simulink model "DateTimeAssemble_test"  (R2013a)
settings: Solver=ode3  StartTime=0.0  StopTime=200  FixedStep=0.001  RelTol=1e-3
libraries: simulink_extras x2, PTC_MBDS_LIB x1
settings Model: Creator=kyle.willis  LastModifiedBy=kyle.willis
settings OptimizationCC: InlineParams=on

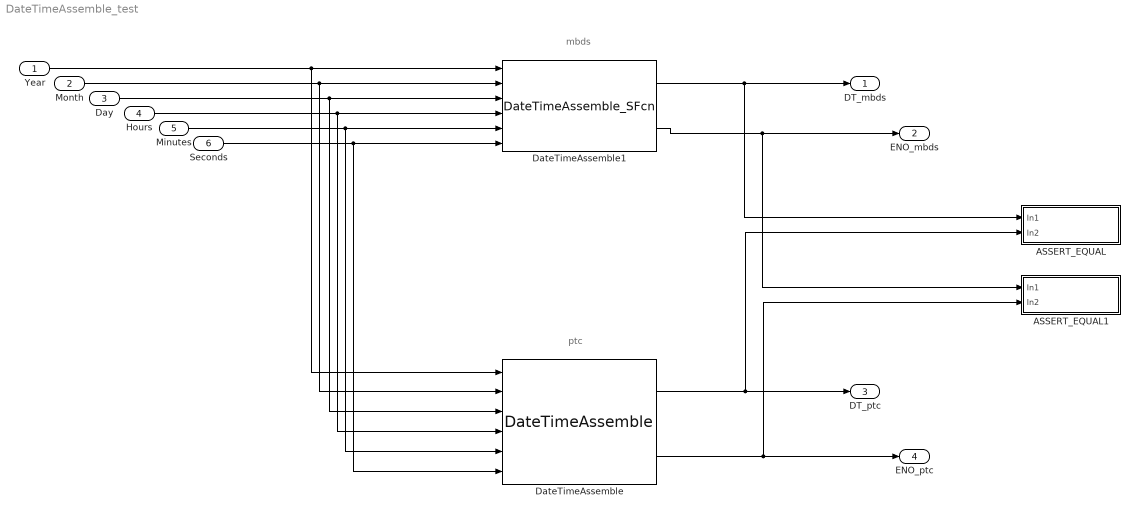
== system DateTimeAssemble_test ==
  note: ptc
  note: mbds
  Year : Inport
  Month : Inport  Port=2
  Day : Inport  Port=3
  Hours : Inport  Port=4
  Minutes : Inport  Port=5
  Seconds : Inport  Port=6
  ASSERT_EQUAL : Subsystem
  ASSERT_EQUAL1 : Subsystem
  DateTimeAssemble : PTC_MBDS_LIB/MBDS Standard Library/Extended Operations/Date & Time Operations/Date & Time Conversions/DateTimeAssemble  ENO_Enabled=on  PTC_MBDS_BlockVersion=5.40  PTC_BlockType=PTC_MBDS_DateTimeAssemble
  DateTimeAssemble1 : S-Function  InitFcn=|  FunctionName=DateTimeAssemble_SFcn  Parameters=boolean(ENO_Enabled)  EnableBusSupport=off  mask(DateTimeAssemble){MBDS_LibraryBlock=on, ENO_Enabled=on, MBDS_BlockVersion=05.41}
      | if(exist('MBDS_BlockCallback', 'file'))
      |    MBDS_BlockCallback('Update', gcb);  
      | end
      mask prompts: MBDS_LibraryBlock "MBDS Library Block"; ENO_Enabled "Show ENO port"; MBDS_BlockVersion "Block version:"
      mask help: Assembles a date_time signal from individual date and time components. The input values are restricted to their ranges (refer to the block help). If an input is out of range the ENO output is set to false.
      mask init:
      | MBDS_BlockCallback('Copy', gcb);     
      | maskdisplay = 'disp(sprintf(''Date Time\nAssemble''))';
      | maskdisplay = [maskdisplay 10 'port_label(''input'', 1, ''Year'')' 10];
      | maskdisplay = [maskdisplay 'port_label(''input'', 2, ''Month'')' 10];
      | maskdisplay = [maskdisplay 'port_label(''input'', 3, ''Day'')' 10];
      | maskdisplay = [maskdisplay 'port_label(''input'', 4, ''Hours'')' 10];
      | maskdisplay = [maskdisplay 'port_label(''input'', 5, ''Minutes'')' 10];
      | maskdisplay = [maskdisplay 'port_label(''input'', 6, ''Seconds'')' 10];
      | maskdisplay = [maskdisplay 'port_label(''output'', 1, ''DT'')' 10];
      | if(ENO_Enabled)
      |     maskdisplay = [maskdisplay 'port_label(''output'', 2, ''ENO'')' 10];
      | end
      | set_param(gcbh, 'maskdisplay', maskdisplay)
      mask Help: eval(['open([workdir(''RT_Dir:''),''\Host\Library\Blockset\Help\'',get_param(gcb,''MaskType''),''.html''])']);
      mask Display:
      | disp(sprintf('Date Time\nAssemble'))
      | port_label('input', 1, 'Year')
      | port_label('input', 2, 'Month')
      | port_label('input', 3, 'Day')
      | port_label('input', 4, 'Hours')
      | port_label('input', 5, 'Minutes')
      | port_label('input', 6, 'Seconds')
      | port_label('output', 1, 'DT')
      | port_label('output', 2, 'ENO')
  DT_mbds : Outport
  ENO_mbds : Outport  Port=2
  DT_ptc : Outport  Port=3
  ENO_ptc : Outport  Port=4
  wires:
  DateTimeAssemble/1 -> ASSERT_EQUAL/2(In2), DT_ptc/1
  DateTimeAssemble/2 -> ASSERT_EQUAL1/2(In2), ENO_ptc/1
  DateTimeAssemble1/1 -> ASSERT_EQUAL/1(In1), DT_mbds/1
  DateTimeAssemble1/2 -> ASSERT_EQUAL1/1(In1), ENO_mbds/1
  Year/1 -> DateTimeAssemble/1, DateTimeAssemble1/1
  Month/1 -> DateTimeAssemble1/2, DateTimeAssemble/2
  Day/1 -> DateTimeAssemble1/3, DateTimeAssemble/3
  Hours/1 -> DateTimeAssemble1/4, DateTimeAssemble/4
  Minutes/1 -> DateTimeAssemble1/5, DateTimeAssemble/5
  Seconds/1 -> DateTimeAssemble1/6, DateTimeAssemble/6

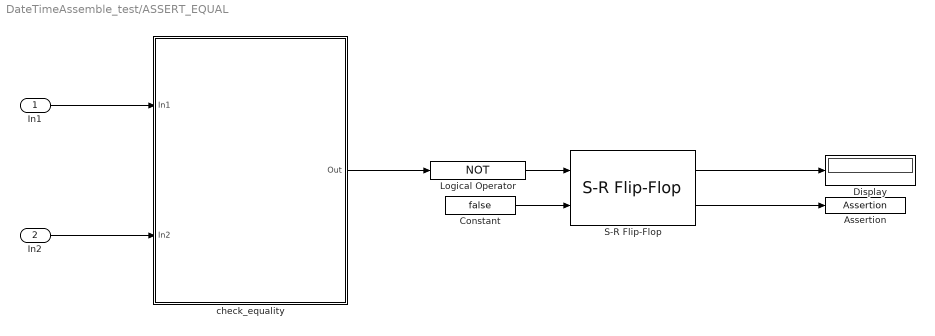
== system DateTimeAssemble_test/ASSERT_EQUAL ==
  In1 : Inport
  In2 : Inport  Port=2
  Assertion : Assertion
  Constant : Constant  Value=false
  Display : Display
  Logical Operator : Logic  Operator=NOT  AllPortsSameDT=off  OutDataTypeStr=boolean
  S-R Flip-Flop : simulink_extras/Flip Flops/S-R Flip-Flop  initial_condition=0
  check_equality : MATLAB Function  TreatAsAtomicUnit=on
  wires:
  S-R Flip-Flop/1 -> Display/1
  check_equality/1(Out) -> Logical Operator/1
  Constant/1 -> S-R Flip-Flop/2
  S-R Flip-Flop/2 -> Assertion/1
  In2/1 -> check_equality/2(In2)
  In1/1 -> check_equality/1(In1)
  Logical Operator/1 -> S-R Flip-Flop/1

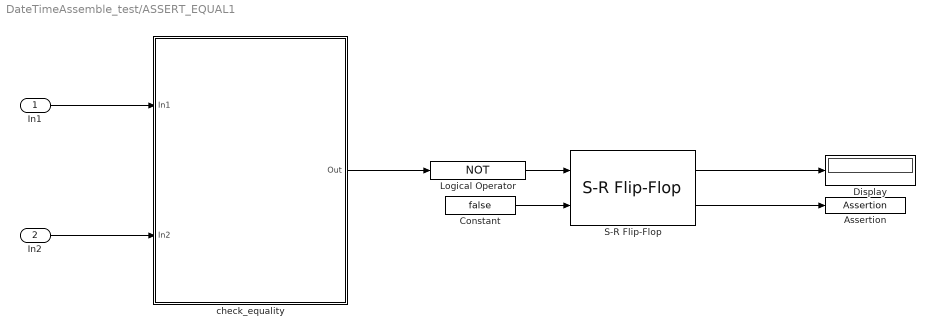
== system DateTimeAssemble_test/ASSERT_EQUAL1 ==
  In1 : Inport
  In2 : Inport  Port=2
  Assertion : Assertion
  Constant : Constant  Value=false
  Display : Display
  Logical Operator : Logic  Operator=NOT  AllPortsSameDT=off  OutDataTypeStr=boolean
  S-R Flip-Flop : simulink_extras/Flip Flops/S-R Flip-Flop  initial_condition=0
  check_equality : MATLAB Function  TreatAsAtomicUnit=on
  wires:
  Logical Operator/1 -> S-R Flip-Flop/1
  In1/1 -> check_equality/1(In1)
  In2/1 -> check_equality/2(In2)
  S-R Flip-Flop/2 -> Assertion/1
  Constant/1 -> S-R Flip-Flop/2
  check_equality/1(Out) -> Logical Operator/1
  S-R Flip-Flop/1 -> Display/1

== matlab function DateTimeAssemble_test/ASSERT_EQUAL1/check_equality ==
  data: In1 input; Out output; In2 input
function Out = check_equality(In1, In2)
%#codegen

Out = isequaln(In1, In2);

end

== matlab function DateTimeAssemble_test/ASSERT_EQUAL/check_equality ==
  data: In1 input; Out output; In2 input
function Out = check_equality(In1, In2)
%#codegen

Out = isequaln(In1, In2);

end
